simulink model "exercise3q1"  (R2023b)
settings: Solver=ode1be  StartTime=0.0  StopTime=10.0  FixedStep=0.001  RelTol=1e-3
undefined symbols (not defined in the file or in its folder): H2
settings Model: Creator=bengo  LastModifiedBy=bengo

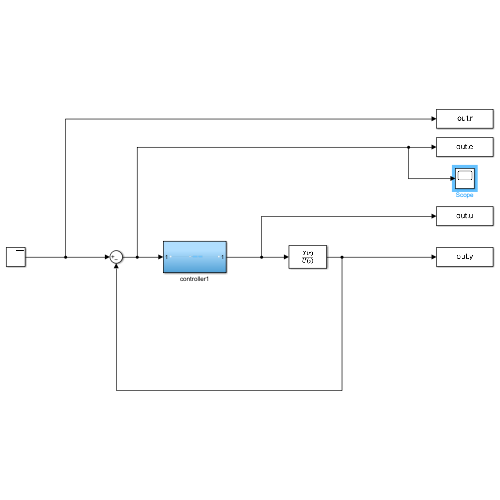
[thumbnail: Simulink's stored preview of the top-level diagram]
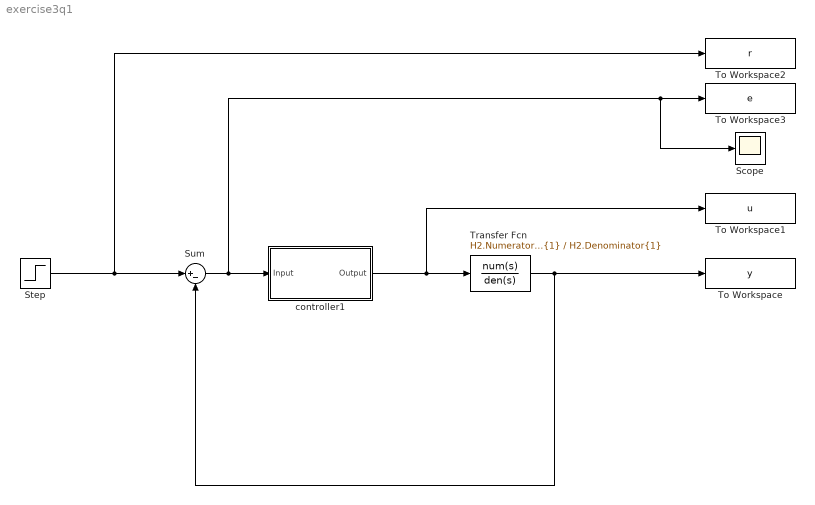
== system exercise3q1 ==
  Scope : Scope
  Step : Step  Time=2  SampleTime=0.001
  Sum : Sum  Inputs=|+-
  To Workspace : ToWorkspace  VariableName=y  SaveFormat=Timeseries  SampleTime=-1
  To Workspace1 : ToWorkspace  VariableName=u  SaveFormat=Timeseries  SampleTime=-1
  To Workspace2 : ToWorkspace  VariableName=r  SaveFormat=Timeseries  SampleTime=-1
  To Workspace3 : ToWorkspace  VariableName=e  SaveFormat=Timeseries  SampleTime=-1
  Transfer Fcn : TransferFcn  Numerator=H2.Numerator{1}  Denominator=H2.Denominator{1}
  controller1 : Subsystem
  wires:
  controller1/1(Output) -> To Workspace1/1, Transfer Fcn/1
  Transfer Fcn/1 -> Sum/2, To Workspace/1
  Step/1 -> To Workspace2/1, Sum/1
  Sum/1 -> Scope/1, To Workspace3/1, controller1/1(Input)

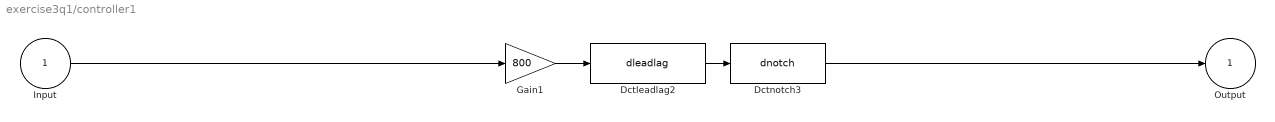
== system exercise3q1/controller1 ==
  Input : Inport
  Dctleadlag2 : S-Function  FunctionName=dleadlag  Parameters=f_num, f_den, 0.001  SFunctionDeploymentMode=off  EnableBusSupport=off  mask(dctools){f_num=10, f_den=90}
      mask prompts: f_num "Zero [Hz]"; f_den "Pole [Hz]"
      mask help: This block implements a discrete time leadlag filter.
      mask Display: disp('DCT leadlag')
  Dctnotch3 : S-Function  FunctionName=dnotch  Parameters=f_num, b_num, f_den, b_den, 0.001  SFunctionDeploymentMode=off  EnableBusSupport=off  mask(dctools){f_num=70, b_num=0.1, f_den=70, b_den=0.2}
      mask prompts: f_num "Zero [Hz]"; b_num "Damping zero [-]"; f_den "Pole [Hz]"; b_den "Damping pole [-]"
      mask help: This block implements a dicrete time 2nd order notch filter.
      mask Display: disp('DCT notch')
  Gain1 : Gain  Gain=800
  Output : Outport
  wires:
  Input/1 -> Gain1/1
  Dctnotch3/1 -> Output/1
  Dctleadlag2/1 -> Dctnotch3/1
  Gain1/1 -> Dctleadlag2/1
